simulink model "fx_v_TxRx_Imprv_final"  (R2020a)
settings: Solver=VariableStepAuto  StartTime=0.0  StopTime=500  RelTol=1e-3
libraries: xbsIndex_r4 x72, simulink x6
settings Model: Creator=RaviM  LastModifiedBy=RaviM

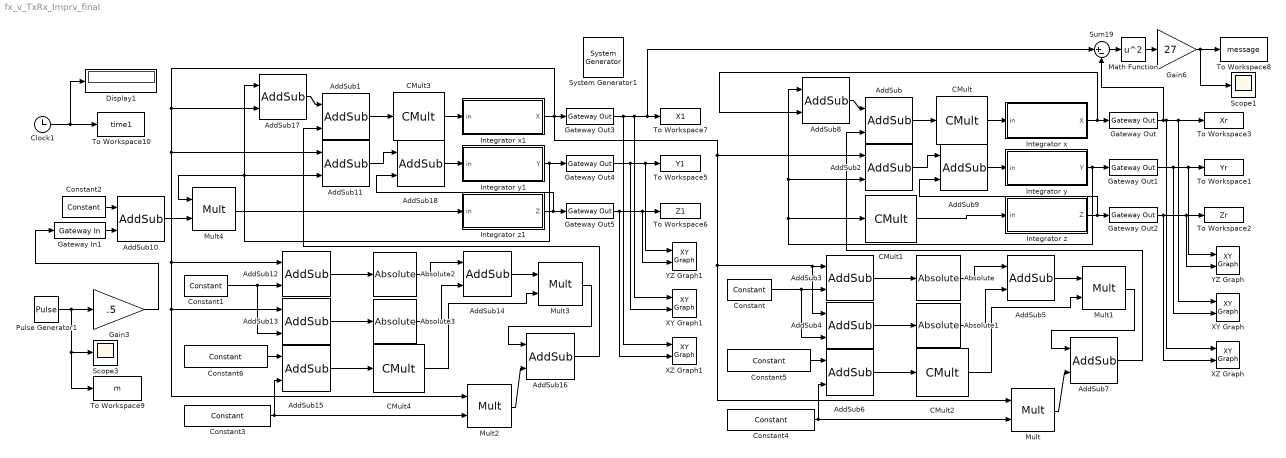
== system fx_v_TxRx_Imprv_final ==
  " System Generator1" : xbsIndex_r4/ System Generator  Tag=genX  xilinxfamily=artix7  part=xc7a100t  speed=-1  package=csg324  synthesis_tool=Vivado  clock_wrapper=Clock Enables  directory=C:/CSULB/Final  proj_type=Vivado  Synth_file=Vivado Synthesis Defaults  Impl_file=Vivado Implementation Defaults  testbench=off  simulink_period=1/100  sysclk_period=100  dcm_input_clock_period=10  incr_netlist=off  trim_vbits=Everywhere in SubSystem  dbl_ovrd=According to Block Masks  core_generation=According to Block Masks  run_coregen=off  deprecated_control=off  eval_field=0  block_type=sysgen
  Absolute{,1..3} (4 alike) : xbsIndex_r4/Absolute  precision=User Defined  arith_type="Signed  (2's comp)"  n_bits=32  bin_pt=24  quantization=Truncate  overflow=Wrap  en=off  latency=0  dbl_ovrd=off  block_type=abs
  AddSub{,1..2,4..6,8,10..11,13..15,17} (13 alike) : xbsIndex_r4/AddSub  mode=Subtraction  use_carryin=off  use_carryout=off  en=off  latency=0  precision=User Defined  arith_type="Signed  (2's comp)"  n_bits=32  bin_pt=24  quantization=Truncate  overflow=Wrap  use_behavioral_HDL=off  hw_selection=DSP48  pipelined=off  dbl_ovrd=off  block_type=addsub
  AddSub{3,7,9,12,16,18} (6 alike) : xbsIndex_r4/AddSub  mode=Addition  use_carryin=off  use_carryout=off  en=off  latency=0  precision=User Defined  arith_type="Signed  (2's comp)"  n_bits=32  bin_pt=24  quantization=Truncate  overflow=Wrap  use_behavioral_HDL=off  hw_selection=DSP48  pipelined=off  dbl_ovrd=off  block_type=addsub
  CMult : xbsIndex_r4/CMult  const=15.8  gui_display_data_type=Fixed-point  const_n_bits=32  const_bin_pt=24  float_type=Single  exp_bits=8  fraction_bits=24  en=off  latency=0  precision=User Defined  arith_type="Signed  (2's comp)"  n_bits=32  bin_pt=24  quantization=Truncate  overflow=Wrap  use_behavioral_HDL=off  mem_type=Distributed RAM  pipeline=off  dbl_ovrd=off  block_type=cmult
  CMult1 : xbsIndex_r4/CMult  const=-36  gui_display_data_type=Fixed-point  const_n_bits=32  const_bin_pt=24  float_type=Single  exp_bits=8  fraction_bits=24  en=off  latency=0  precision=User Defined  arith_type="Signed  (2's comp)"  n_bits=32  bin_pt=24  quantization=Truncate  overflow=Wrap  use_behavioral_HDL=off  mem_type=Distributed RAM  pipeline=off  dbl_ovrd=off  block_type=cmult
  CMult2 : xbsIndex_r4/CMult  const=1  gui_display_data_type=Fixed-point  const_n_bits=32  const_bin_pt=24  float_type=Single  exp_bits=8  fraction_bits=24  en=off  latency=0  precision=User Defined  arith_type="Signed  (2's comp)"  n_bits=32  bin_pt=24  quantization=Truncate  overflow=Wrap  use_behavioral_HDL=off  mem_type=Distributed RAM  pipeline=off  dbl_ovrd=off  block_type=cmult
  CMult3 : xbsIndex_r4/CMult  const=15.8  gui_display_data_type=Fixed-point  const_n_bits=32  const_bin_pt=24  float_type=Single  exp_bits=8  fraction_bits=24  en=off  latency=0  precision=User Defined  arith_type="Signed  (2's comp)"  n_bits=32  bin_pt=24  quantization=Truncate  overflow=Wrap  use_behavioral_HDL=off  mem_type=Distributed RAM  pipeline=off  dbl_ovrd=off  block_type=cmult
  CMult4 : xbsIndex_r4/CMult  const=1  gui_display_data_type=Fixed-point  const_n_bits=32  const_bin_pt=24  float_type=Single  exp_bits=8  fraction_bits=24  en=off  latency=0  precision=User Defined  arith_type="Signed  (2's comp)"  n_bits=32  bin_pt=24  quantization=Truncate  overflow=Wrap  use_behavioral_HDL=off  mem_type=Distributed RAM  pipeline=off  dbl_ovrd=off  block_type=cmult
  Clock1 : Clock
  Constant : xbsIndex_r4/Constant  const=1.0  gui_display_data_type=Fixed-point  arith_type=Signed (2's comp)  n_bits=32  bin_pt=24  preci_type=Single  exp_width=8  frac_width=24  explicit_period=on  period=1  equ=P=C  opselect=C  inp2=PCIN>>17  opr=+  inp1=P  carry=CIN  dbl_ovrd=off  block_type=constant
  Constant1 : xbsIndex_r4/Constant  const=1.0  gui_display_data_type=Fixed-point  arith_type=Signed (2's comp)  n_bits=32  bin_pt=24  preci_type=Single  exp_width=8  frac_width=24  explicit_period=on  period=1  equ=P=C  opselect=C  inp2=PCIN>>17  opr=+  inp1=P  carry=CIN  dbl_ovrd=off  block_type=constant
  Constant2 : xbsIndex_r4/Constant  const=-35.5  gui_display_data_type=Fixed-point  arith_type=Signed (2's comp)  n_bits=32  bin_pt=24  preci_type=Single  exp_width=8  frac_width=24  explicit_period=on  period=1  equ=P=C  opselect=C  inp2=PCIN>>17  opr=+  inp1=P  carry=CIN  dbl_ovrd=off  block_type=constant
  Constant3 : xbsIndex_r4/Constant  const=-5/7  gui_display_data_type=Fixed-point  arith_type=Signed (2's comp)  n_bits=32  bin_pt=24  preci_type=Single  exp_width=8  frac_width=24  explicit_period=on  period=1  equ=P=C  opselect=C  inp2=PCIN>>17  opr=+  inp1=P  carry=CIN  dbl_ovrd=off  block_type=constant
  Constant4 : xbsIndex_r4/Constant  const=-5/7  gui_display_data_type=Fixed-point  arith_type=Signed (2's comp)  n_bits=32  bin_pt=24  preci_type=Single  exp_width=8  frac_width=24  explicit_period=on  period=1  equ=P=C  opselect=C  inp2=PCIN>>17  opr=+  inp1=P  carry=CIN  dbl_ovrd=off  block_type=constant
  Constant5 : xbsIndex_r4/Constant  const=-9/7  gui_display_data_type=Fixed-point  arith_type=Signed (2's comp)  n_bits=32  bin_pt=24  preci_type=Single  exp_width=8  frac_width=24  explicit_period=on  period=1  equ=P=C  opselect=C  inp2=PCIN>>17  opr=+  inp1=P  carry=CIN  dbl_ovrd=off  block_type=constant
  Constant6 : xbsIndex_r4/Constant  const=-9/7  gui_display_data_type=Fixed-point  arith_type=Signed (2's comp)  n_bits=32  bin_pt=24  preci_type=Single  exp_width=8  frac_width=24  explicit_period=on  period=1  equ=P=C  opselect=C  inp2=PCIN>>17  opr=+  inp1=P  carry=CIN  dbl_ovrd=off  block_type=constant
  Display1 : Display
      settings: Decimation=5
  Gain3 : Gain  Gain=.5
  Gain6 : Gain  Gain=27
  Gateway In1 : xbsIndex_r4/Gateway In  gui_display_data_type=Fixed-point  arith_type="Signed  (2's comp)"  n_bits=16  bin_pt=14  preci_type=Single  exp_width=8  frac_width=24  rows=1  columns=1  quantization="Round  (unbiased: +/- Inf)"  overflow=Saturate  period=1  UseAsADC=off  ADCChannel='1'  interface=None  automatic_assignment=on  address_offset=hex2dec('00')  intf_name=''  intf_description=''  default_value=0  timing_constraint=None  locs_specified=off  LOCs={}  io_standard={}  inherit_from_input=off  hdl_port=on  dbl_ovrd=off  block_type=gatewayin
  Gateway Out{,1..5} (6 alike) : xbsIndex_r4/Gateway Out  inherit_from_input=off  hdl_port=on  rows=1  columns=1  UseAsDAC=off  DACChannel='1'  interface=None  automatic_assignment=on  address_offset=hex2dec('00')  intf_name=''  intf_description=''  timing_constraint=None  locs_specified=off  LOCs={}  io_standard={}  block_type=gatewayout
  Integrator x : Subsystem
  Integrator x1 : Subsystem
  Integrator y : Subsystem
  Integrator y1 : Subsystem
  Integrator z : Subsystem
  Integrator z1 : Subsystem
  Math Function : Math  Operator=square  SignedPower=on  SaturateOnIntegerOverflow=on
  Mult{,1..4} (5 alike) : xbsIndex_r4/Mult  precision=User Defined  arith_type="Signed  (2's comp)"  n_bits=32  bin_pt=24  quantization=Truncate  overflow=Wrap  en=off  latency=0  use_behavioral_HDL=off  opt=Speed  use_embedded=on  optimum_pipeline=off  pipeline=on  dbl_ovrd=off  use_rpm=on  placement_style=Triangular  block_type=mult
  Pulse Generator1 : DiscretePulseGenerator  PulseType=Time based  Amplitude=5  Period=100  PulseWidth=50  PhaseDelay=50
  Scope1 : Scope
  Scope3 : Scope
  Sum19 : Sum  Inputs=|+-
  To Workspace1 : ToWorkspace  VariableName=Yr  SaveFormat=Timeseries  SampleTime=-1
  To Workspace10 : ToWorkspace  VariableName=time1  SampleTime=-1
  To Workspace2 : ToWorkspace  VariableName=Zr  SaveFormat=Timeseries  SampleTime=-1
  To Workspace3 : ToWorkspace  VariableName=Xr  SaveFormat=Timeseries  SampleTime=-1
  To Workspace5 : ToWorkspace  VariableName=Y1  SaveFormat=Timeseries  SampleTime=-1
  To Workspace6 : ToWorkspace  VariableName=Z1  SaveFormat=Timeseries  SampleTime=-1
  To Workspace7 : ToWorkspace  VariableName=X1  SaveFormat=Timeseries  SampleTime=-1
  To Workspace8 : ToWorkspace  VariableName=message  SampleTime=-1
  To Workspace9 : ToWorkspace  VariableName=m  SampleTime=-1
  XY Graph : simulink/Sinks/XY Graph  xmin=-20  xmax=20  ymin=-20  ymax=20  st=-1
  XY Graph1 : simulink/Sinks/XY Graph  xmin=-20  xmax=20  ymin=-20  ymax=20  st=-1
  XZ Graph : simulink/Sinks/XY Graph  xmin=-20  xmax=20  ymin=-20  ymax=20  st=-1
  XZ Graph1 : simulink/Sinks/XY Graph  xmin=-20  xmax=20  ymin=-20  ymax=20  st=-1
  YZ Graph : simulink/Sinks/XY Graph  xmin=-20  xmax=20  ymin=-20  ymax=20  st=-1
  YZ Graph1 : simulink/Sinks/XY Graph  xmin=-20  xmax=20  ymin=-20  ymax=20  st=-1
  wires:
  Integrator x1/1(X) -> AddSub2/1, AddSub4/1, AddSub3/1, Mult/1, AddSub12/1, AddSub13/1, Mult2/1, AddSub11/1, AddSub17/2, Gateway Out3/1
  Gain6/1 -> Scope1/1, To Workspace8/1
  Gateway Out1/1 -> To Workspace1/1, YZ Graph/1, XY Graph/2
  Integrator z/1(Z) -> Gateway Out2/1, AddSub9/2
  Gateway Out2/1 -> To Workspace2/1, YZ Graph/2, XZ Graph/2
  Gateway Out/1 -> To Workspace3/1, XY Graph/1, XZ Graph/1, Sum19/2
  Absolute1/1 -> AddSub5/2
  CMult1/1 -> Integrator z/1(in)
  AddSub/1 -> CMult/1
  Sum19/1 -> Math Function/1
  Math Function/1 -> Gain6/1
  Constant5/1 -> AddSub6/1
  Constant/1 -> AddSub4/2, AddSub3/2
  CMult/1 -> Integrator x/1(in)
  AddSub8/1 -> AddSub/1
  AddSub9/1 -> Integrator y/1(in)
  AddSub4/1 -> Absolute1/1
  Integrator x/1(X) -> AddSub8/2, Gateway Out/1
  AddSub2/1 -> AddSub9/1
  AddSub6/1 -> CMult2/1
  Mult/1 -> AddSub7/2
  Constant4/1 -> AddSub6/2, Mult/2
  Absolute/1 -> AddSub5/1
  Mult1/1 -> AddSub7/1
  CMult2/1 -> Mult1/2
  AddSub3/1 -> Absolute/1
  Integrator y/1(Y) -> Gateway Out1/1, AddSub8/1, AddSub2/2, CMult1/1
  AddSub7/1 -> AddSub/2
  AddSub5/1 -> Mult1/1
  Gateway Out5/1 -> To Workspace6/1, YZ Graph1/2, XZ Graph1/2
  Constant6/1 -> AddSub15/1
  Constant1/1 -> AddSub13/2, AddSub12/2
  Mult3/1 -> AddSub16/1
  CMult4/1 -> Mult3/2
  AddSub18/1 -> Integrator y1/1(in)
  Constant2/1 -> AddSub10/1
  Clock1/1 -> Display1/1, To Workspace10/1
  Pulse Generator1/1 -> To Workspace9/1, Scope3/1, Gain3/1
  Absolute3/1 -> AddSub14/2
  Gateway In1/1 -> AddSub10/2
  Gateway Out3/1 -> Sum19/1, To Workspace7/1, XY Graph1/1, XZ Graph1/1
  Gateway Out4/1 -> To Workspace5/1, YZ Graph1/1, XY Graph1/2
  AddSub10/1 -> Mult4/2
  Integrator z1/1(Z) -> Gateway Out5/1, AddSub18/2
  AddSub12/1 -> Absolute2/1
  AddSub16/1 -> AddSub1/2
  Gain3/1 -> Gateway In1/1
  Integrator y1/1(Y) -> Gateway Out4/1, AddSub17/1, Mult4/1, AddSub11/2
  AddSub17/1 -> AddSub1/1
  AddSub11/1 -> AddSub18/1
  Mult2/1 -> AddSub16/2
  Constant3/1 -> AddSub15/2, Mult2/2
  AddSub13/1 -> Absolute3/1
  AddSub15/1 -> CMult4/1
  AddSub14/1 -> Mult3/1
  Absolute2/1 -> AddSub14/1
  AddSub1/1 -> CMult3/1
  Mult4/1 -> Integrator z1/1(in)
  CMult3/1 -> Integrator x1/1(in)

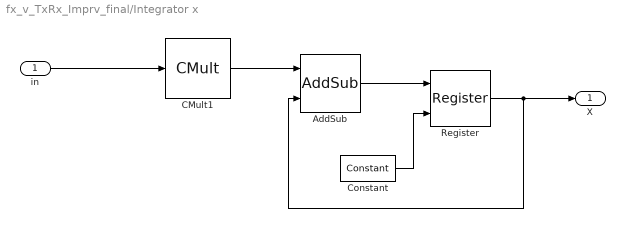
== system fx_v_TxRx_Imprv_final/Integrator x ==
  in : Inport
  AddSub : xbsIndex_r4/AddSub  mode=Addition  use_carryin=off  use_carryout=off  en=off  latency=0  precision=User Defined  arith_type="Signed  (2's comp)"  n_bits=32  bin_pt=24  quantization=Truncate  overflow=Wrap  use_behavioral_HDL=off  hw_selection=DSP48  pipelined=off  dbl_ovrd=off  block_type=addsub
  CMult1 : xbsIndex_r4/CMult  const=0.01  gui_display_data_type=Fixed-point  const_n_bits=32  const_bin_pt=24  float_type=Single  exp_bits=8  fraction_bits=24  en=off  latency=0  precision=User Defined  arith_type="Signed  (2's comp)"  n_bits=32  bin_pt=24  quantization=Truncate  overflow=Wrap  use_behavioral_HDL=off  mem_type=Distributed RAM  pipeline=off  dbl_ovrd=off  block_type=cmult
  Constant : xbsIndex_r4/Constant  const=0  gui_display_data_type=Boolean  arith_type=Boolean  n_bits=16  bin_pt=14  preci_type=Single  exp_width=8  frac_width=24  explicit_period=on  period=0.01  equ=P=C  opselect=C  inp2=PCIN>>17  opr=+  inp1=P  carry=CIN  dbl_ovrd=off  block_type=constant
  Register : xbsIndex_r4/Register  init=0.1  rst=on  en=off  dbl_ovrd=off  block_type=register
      settings: block_version=11.1
  X : Outport  SampleTime=0.01
  wires:
  CMult1/1 -> AddSub/1
  AddSub/1 -> Register/1
  Register/1 -> X/1, AddSub/2
  in/1 -> CMult1/1
  Constant/1 -> Register/2

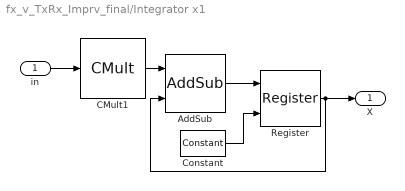
== system fx_v_TxRx_Imprv_final/Integrator x1 ==
  in : Inport
  AddSub : xbsIndex_r4/AddSub  mode=Addition  use_carryin=off  use_carryout=off  en=off  latency=0  precision=User Defined  arith_type="Signed  (2's comp)"  n_bits=32  bin_pt=24  quantization=Truncate  overflow=Wrap  use_behavioral_HDL=off  hw_selection=DSP48  pipelined=off  dbl_ovrd=off  block_type=addsub
  CMult1 : xbsIndex_r4/CMult  const=0.01  gui_display_data_type=Fixed-point  const_n_bits=32  const_bin_pt=24  float_type=Single  exp_bits=8  fraction_bits=24  en=off  latency=0  precision=User Defined  arith_type="Signed  (2's comp)"  n_bits=32  bin_pt=24  quantization=Truncate  overflow=Wrap  use_behavioral_HDL=off  mem_type=Distributed RAM  pipeline=off  dbl_ovrd=off  block_type=cmult
  Constant : xbsIndex_r4/Constant  const=0  gui_display_data_type=Boolean  arith_type=Boolean  n_bits=16  bin_pt=14  preci_type=Single  exp_width=8  frac_width=24  explicit_period=on  period=0.01  equ=P=C  opselect=C  inp2=PCIN>>17  opr=+  inp1=P  carry=CIN  dbl_ovrd=off  block_type=constant
  Register : xbsIndex_r4/Register  init=0.1  rst=on  en=off  dbl_ovrd=off  block_type=register
      settings: block_version=11.1
  X : Outport  SampleTime=0.01
  wires:
  CMult1/1 -> AddSub/1
  AddSub/1 -> Register/1
  Register/1 -> X/1, AddSub/2
  in/1 -> CMult1/1
  Constant/1 -> Register/2

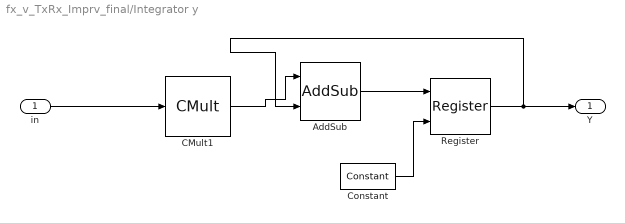
== system fx_v_TxRx_Imprv_final/Integrator y ==
  in : Inport
  AddSub : xbsIndex_r4/AddSub  mode=Addition  use_carryin=off  use_carryout=off  en=off  latency=0  precision=User Defined  arith_type="Signed  (2's comp)"  n_bits=32  bin_pt=24  quantization=Truncate  overflow=Wrap  use_behavioral_HDL=off  hw_selection=DSP48  pipelined=off  dbl_ovrd=off  block_type=addsub
  CMult1 : xbsIndex_r4/CMult  const=0.01  gui_display_data_type=Fixed-point  const_n_bits=32  const_bin_pt=24  float_type=Single  exp_bits=8  fraction_bits=24  en=off  latency=0  precision=User Defined  arith_type="Signed  (2's comp)"  n_bits=32  bin_pt=24  quantization=Truncate  overflow=Wrap  use_behavioral_HDL=off  mem_type=Distributed RAM  pipeline=off  dbl_ovrd=off  block_type=cmult
  Constant : xbsIndex_r4/Constant  const=0  gui_display_data_type=Boolean  arith_type=Boolean  n_bits=16  bin_pt=14  preci_type=Single  exp_width=8  frac_width=24  explicit_period=on  period=0.01  equ=P=C  opselect=C  inp2=PCIN>>17  opr=+  inp1=P  carry=CIN  dbl_ovrd=off  block_type=constant
  Register : xbsIndex_r4/Register  init=0.1  rst=on  en=off  dbl_ovrd=off  block_type=register
  Y : Outport
  wires:
  in/1 -> CMult1/1
  AddSub/1 -> Register/1
  Constant/1 -> Register/2
  CMult1/1 -> AddSub/1
  Register/1 -> Y/1, AddSub/2

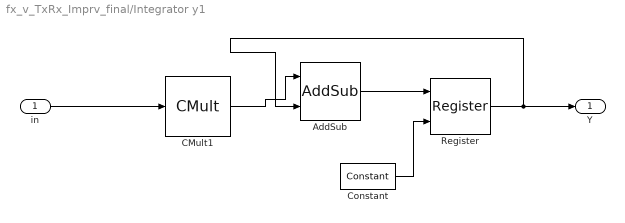
== system fx_v_TxRx_Imprv_final/Integrator y1 ==
  in : Inport
  AddSub : xbsIndex_r4/AddSub  mode=Addition  use_carryin=off  use_carryout=off  en=off  latency=0  precision=User Defined  arith_type="Signed  (2's comp)"  n_bits=32  bin_pt=24  quantization=Truncate  overflow=Wrap  use_behavioral_HDL=off  hw_selection=DSP48  pipelined=off  dbl_ovrd=off  block_type=addsub
  CMult1 : xbsIndex_r4/CMult  const=0.01  gui_display_data_type=Fixed-point  const_n_bits=32  const_bin_pt=24  float_type=Single  exp_bits=8  fraction_bits=24  en=off  latency=0  precision=User Defined  arith_type="Signed  (2's comp)"  n_bits=32  bin_pt=24  quantization=Truncate  overflow=Wrap  use_behavioral_HDL=off  mem_type=Distributed RAM  pipeline=off  dbl_ovrd=off  block_type=cmult
  Constant : xbsIndex_r4/Constant  const=0  gui_display_data_type=Boolean  arith_type=Boolean  n_bits=16  bin_pt=14  preci_type=Single  exp_width=8  frac_width=24  explicit_period=on  period=0.01  equ=P=C  opselect=C  inp2=PCIN>>17  opr=+  inp1=P  carry=CIN  dbl_ovrd=off  block_type=constant
  Register : xbsIndex_r4/Register  init=0.1  rst=on  en=off  dbl_ovrd=off  block_type=register
  Y : Outport
  wires:
  in/1 -> CMult1/1
  AddSub/1 -> Register/1
  Constant/1 -> Register/2
  CMult1/1 -> AddSub/1
  Register/1 -> Y/1, AddSub/2

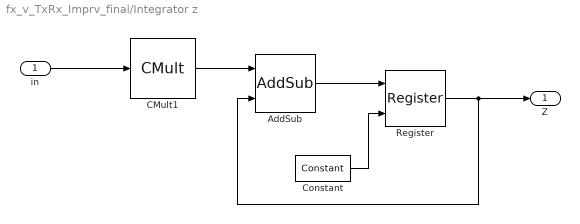
== system fx_v_TxRx_Imprv_final/Integrator z ==
  in : Inport
  AddSub : xbsIndex_r4/AddSub  mode=Addition  use_carryin=off  use_carryout=off  en=off  latency=0  precision=User Defined  arith_type="Signed  (2's comp)"  n_bits=32  bin_pt=24  quantization=Truncate  overflow=Wrap  use_behavioral_HDL=off  hw_selection=DSP48  pipelined=off  dbl_ovrd=off  block_type=addsub
  CMult1 : xbsIndex_r4/CMult  const=0.01  gui_display_data_type=Fixed-point  const_n_bits=32  const_bin_pt=24  float_type=Single  exp_bits=8  fraction_bits=24  en=off  latency=0  precision=User Defined  arith_type="Signed  (2's comp)"  n_bits=32  bin_pt=24  quantization=Truncate  overflow=Wrap  use_behavioral_HDL=off  mem_type=Distributed RAM  pipeline=off  dbl_ovrd=off  block_type=cmult
  Constant : xbsIndex_r4/Constant  const=0  gui_display_data_type=Boolean  arith_type=Boolean  n_bits=16  bin_pt=14  preci_type=Single  exp_width=8  frac_width=24  explicit_period=on  period=0.01  equ=P=C  opselect=C  inp2=PCIN>>17  opr=+  inp1=P  carry=CIN  dbl_ovrd=off  block_type=constant
  Register : xbsIndex_r4/Register  init=0.1  rst=on  en=off  dbl_ovrd=off  block_type=register
  Z : Outport
  wires:
  in/1 -> CMult1/1
  AddSub/1 -> Register/1
  Constant/1 -> Register/2
  CMult1/1 -> AddSub/1
  Register/1 -> Z/1, AddSub/2

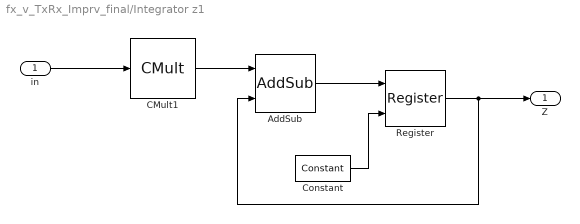
== system fx_v_TxRx_Imprv_final/Integrator z1 ==
  in : Inport
  AddSub : xbsIndex_r4/AddSub  mode=Addition  use_carryin=off  use_carryout=off  en=off  latency=0  precision=User Defined  arith_type="Signed  (2's comp)"  n_bits=32  bin_pt=24  quantization=Truncate  overflow=Wrap  use_behavioral_HDL=off  hw_selection=DSP48  pipelined=off  dbl_ovrd=off  block_type=addsub
  CMult1 : xbsIndex_r4/CMult  const=0.01  gui_display_data_type=Fixed-point  const_n_bits=32  const_bin_pt=24  float_type=Single  exp_bits=8  fraction_bits=24  en=off  latency=0  precision=User Defined  arith_type="Signed  (2's comp)"  n_bits=32  bin_pt=24  quantization=Truncate  overflow=Wrap  use_behavioral_HDL=off  mem_type=Distributed RAM  pipeline=off  dbl_ovrd=off  block_type=cmult
  Constant : xbsIndex_r4/Constant  const=0  gui_display_data_type=Boolean  arith_type=Boolean  n_bits=16  bin_pt=14  preci_type=Single  exp_width=8  frac_width=24  explicit_period=on  period=0.01  equ=P=C  opselect=C  inp2=PCIN>>17  opr=+  inp1=P  carry=CIN  dbl_ovrd=off  block_type=constant
  Register : xbsIndex_r4/Register  init=0.1  rst=on  en=off  dbl_ovrd=off  block_type=register
  Z : Outport
  wires:
  in/1 -> CMult1/1
  AddSub/1 -> Register/1
  Constant/1 -> Register/2
  CMult1/1 -> AddSub/1
  Register/1 -> Z/1, AddSub/2
